simulink model "paper3"  (R2022a)
settings: Solver=VariableStepAuto  StartTime=0.0  StopTime=50  RelTol=1e-3
settings Model: Creator=mudit  LastModifiedBy=mudit

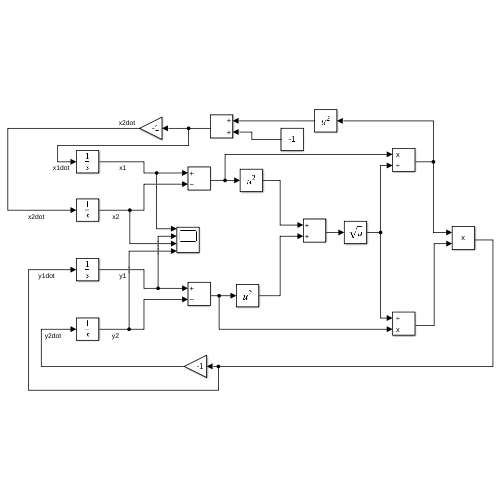
[thumbnail: Simulink's stored preview of the top-level diagram]
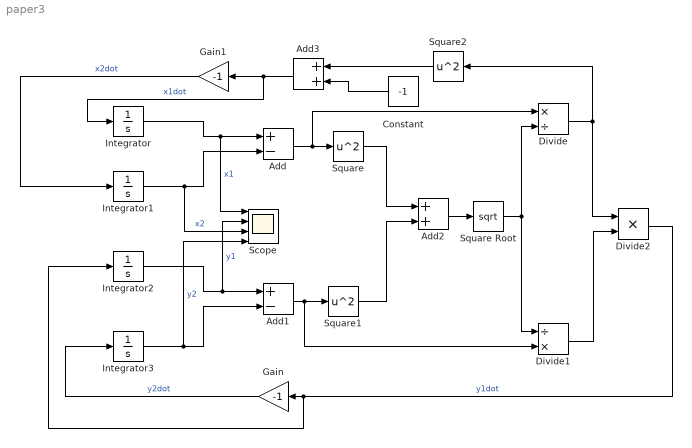
== system paper3 ==
  Add : Sum  Inputs=+-
  Add1 : Sum  Inputs=+-
  Add2 : Sum
  Add3 : Sum
  Constant : Constant  Value=-1
  Divide : Product  Inputs=*/
  Divide1 : Product  Inputs=/*
  Divide2 : Product  Inputs=**
  Gain : Gain  Gain=-1
  Gain1 : Gain  Gain=-1
  Integrator : Integrator  InitialCondition=-1
  Integrator1 : Integrator  InitialCondition=3
  Integrator2 : Integrator  InitialCondition=10
  Integrator3 : Integrator  InitialCondition=1
  Scope : Scope  NumInputPorts=4
  Square : Math  Operator=square
  Square Root : Sqrt
  Square1 : Math  Operator=square
  Square2 : Math  Operator=square
  wires:
  Add3/1 -> Integrator/1, Gain1/1  "x1dot"
  Divide2/1 -> Integrator2/1, Gain/1  "y1dot"
  Gain/1 -> Integrator3/1  "y2dot"
  Integrator/1 -> Scope/1, Add/1  "x1"
  Integrator1/1 -> Scope/3, Add/2  "x2"
  Integrator2/1 -> Scope/2, Add1/1  "y1"
  Integrator3/1 -> Add1/2, Scope/4  "y2"
  Add/1 -> Divide/1, Square/1
  Add1/1 -> Divide1/2, Square1/1
  Square/1 -> Add2/1
  Square1/1 -> Add2/2
  Add2/1 -> Square Root/1
  Square Root/1 -> Divide/2, Divide1/1
  Divide/1 -> Divide2/1, Square2/1
  Divide1/1 -> Divide2/2
  Square2/1 -> Add3/1
  Constant/1 -> Add3/2
  Gain1/1 -> Integrator1/1  "x2dot"
